simulink model "MySelectorCtrlMapping_RTW"  (R2022a)
settings: Solver=ode1  StartTime=0.0  StopTime=inf  FixedStep=0.001  RelTol=1e-3
PreLoadFcn:
  | vehicle = 'Car'; if ~length(which('cmself')), cmenv; end
  | MySelectorCtrlMapping_RTW_bus
InitFcn:
  | vehicle = 'Car'; if ~length(which('cmself')), cmenv; end
  | MySelectorCtrlMapping_RTW_bus
libraries: simulink x2
Description:
  | CarMaker Plug-in Model Target
settings Model: Creator=IPG  LastModifiedBy=IPG
settings DebuggingCC: UnconnectedInputMsg=warning  UnconnectedOutputMsg=warning  UnconnectedLineMsg=warning
settings RTWCC: Description=CarMaker Plug-in Model Target  SystemTargetFile=CarMaker.tlc  TemplateMakefile=CarMaker_unix-win64.tmf  DLArmComputeVersion=19.05
settings CodeAppCC: MaxIdLength=127
settings STFCustomTargetCC: TargetLangStandard=C99 (ISO)  CombineOutputUpdateFcns=on  MatFileLogging=on  CodeInterfacePackaging=Reusable function  GRTInterface=off  GenerateAllocFcn=on  SystemTargetFile=CarMaker.tlc
settings GRTTargetCC: ParMdlRefBuildCompliant=off  CompOptLevelCompliant=off  ConcurrentExecutionCompliant=off  CodeInterfacePackaging=Reusable function  CPPClassGenCompliant=off  GenerateAllocFcn=on  UseToolchainInfoCompliant=off

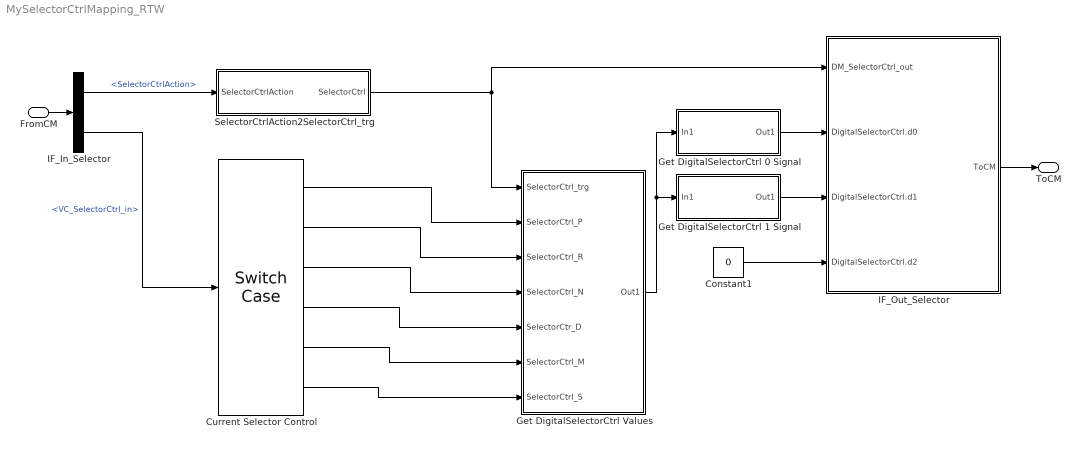
== system MySelectorCtrlMapping_RTW ==
  FromCM : Inport  OutDataTypeStr=Bus: cmSelectorCtrlMappingIn
  Constant1 : Constant  Value=0
  Current Selector Control : SwitchCase  CaseConditions={-9, -1, 0, 1, 2, 3}  ShowDefaultCase=off
  Get DigitalSelectorCtrl 0 Signal : Subsystem
  Get DigitalSelectorCtrl 1 Signal : Subsystem
  Get DigitalSelectorCtrl Values : Subsystem
  IF_In_Selector : BusSelector  OutputSignals=SelectorCtrlAction,VC_SelectorCtrl_in
  IF_Out_Selector : Subsystem  mask(Signal Selection){}
      mask help: Signal Selection Block
      settings: OpenFcn=cmSignalSelect('SignalSelection_CB',gcb)
  SelectorCtrlAction2SelectorCtrl_trg : Subsystem
  ToCM : Outport  OutDataTypeStr=Bus: cmSelectorCtrlMappingOut
  wires:
  FromCM/1 -> IF_In_Selector/1
  IF_Out_Selector/1(ToCM) -> ToCM/1
  Current Selector Control/6 -> Get DigitalSelectorCtrl Values/7(SelectorCtrl_S)
  IF_In_Selector/1 -> SelectorCtrlAction2SelectorCtrl_trg/1(SelectorCtrlAction)  "<SelectorCtrlAction>"
  Current Selector Control/2 -> Get DigitalSelectorCtrl Values/3(SelectorCtrl_R)
  Get DigitalSelectorCtrl 0 Signal/1(Out1) -> IF_Out_Selector/2(DigitalSelectorCtrl.d0)
  Get DigitalSelectorCtrl 1 Signal/1(Out1) -> IF_Out_Selector/3(DigitalSelectorCtrl.d1)
  Current Selector Control/3 -> Get DigitalSelectorCtrl Values/4(SelectorCtrl_N)
  SelectorCtrlAction2SelectorCtrl_trg/1(SelectorCtrl) -> IF_Out_Selector/1(DM_SelectorCtrl_out), Get DigitalSelectorCtrl Values/1(SelectorCtrl_trg)
  Current Selector Control/5 -> Get DigitalSelectorCtrl Values/6(SelectorCtrl_M)
  Current Selector Control/1 -> Get DigitalSelectorCtrl Values/2(SelectorCtrl_P)
  Constant1/1 -> IF_Out_Selector/4(DigitalSelectorCtrl.d2)
  Current Selector Control/4 -> Get DigitalSelectorCtrl Values/5(SelectorCtr_D)
  IF_In_Selector/2 -> Current Selector Control/1  "<VC_SelectorCtrl_in>"
  Get DigitalSelectorCtrl Values/1(Out1) -> Get DigitalSelectorCtrl 1 Signal/1(In1), Get DigitalSelectorCtrl 0 Signal/1(In1)

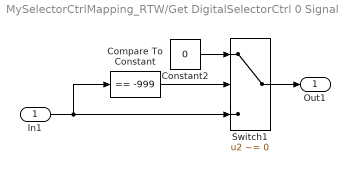
== system MySelectorCtrlMapping_RTW/Get DigitalSelectorCtrl 0 Signal ==
  In1 : Inport
  Compare To Constant : simulink/Logic and Bit Operations/Compare To Constant  relop===  const=-999  OutDataTypeStr=boolean
  Constant2 : Constant  Value=0
  Switch1 : Switch  Criteria=u2 ~= 0  SaturateOnIntegerOverflow=off  InputSameDT=off
  Out1 : Outport
  wires:
  Compare To Constant/1 -> Switch1/2
  Constant2/1 -> Switch1/1
  In1/1 -> Switch1/3, Compare To Constant/1
  Switch1/1 -> Out1/1

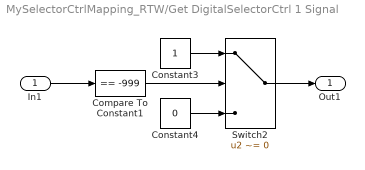
== system MySelectorCtrlMapping_RTW/Get DigitalSelectorCtrl 1 Signal ==
  In1 : Inport
  Compare To Constant1 : simulink/Logic and Bit Operations/Compare To Constant  relop===  const=-999  OutDataTypeStr=boolean
  Constant3 : Constant
  Constant4 : Constant  Value=0
  Switch2 : Switch  Criteria=u2 ~= 0  SaturateOnIntegerOverflow=off  InputSameDT=off
  Out1 : Outport
  wires:
  Compare To Constant1/1 -> Switch2/2
  Constant3/1 -> Switch2/1
  Constant4/1 -> Switch2/3
  In1/1 -> Compare To Constant1/1
  Switch2/1 -> Out1/1

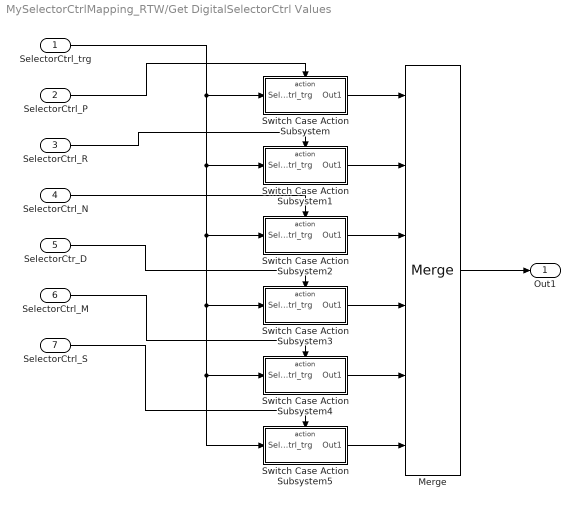
== system MySelectorCtrlMapping_RTW/Get DigitalSelectorCtrl Values ==
  SelectorCtrl_trg : Inport
  SelectorCtrl_P : Inport  Port=2
  SelectorCtrl_R : Inport  Port=3
  SelectorCtrl_N : Inport  Port=4
  SelectorCtr_D : Inport  Port=5
  SelectorCtrl_M : Inport  Port=6
  SelectorCtrl_S : Inport  Port=7
  Merge : Merge  Inputs=6
  Switch Case Action Subsystem : Subsystem  TreatAsAtomicUnit=on
  Switch Case Action Subsystem1 : Subsystem  TreatAsAtomicUnit=on
  Switch Case Action Subsystem2 : Subsystem  TreatAsAtomicUnit=on
  Switch Case Action Subsystem3 : Subsystem  TreatAsAtomicUnit=on
  Switch Case Action Subsystem4 : Subsystem  TreatAsAtomicUnit=on
  Switch Case Action Subsystem5 : Subsystem  TreatAsAtomicUnit=on
  Out1 : Outport
  wires:
  SelectorCtrl_trg/1 -> Switch Case Action Subsystem5/1(SelectorCtrl_trg), Switch Case Action Subsystem4/1(SelectorCtrl_trg), Switch Case Action Subsystem3/1(SelectorCtrl_trg), Switch Case Action Subsystem2/1(SelectorCtrl_trg), Switch Case Action Subsystem1/1(SelectorCtrl_trg), Switch Case Action Subsystem/1(SelectorCtrl_trg)
  SelectorCtrl_R/1 -> Switch Case Action Subsystem1/Action
  SelectorCtrl_N/1 -> Switch Case Action Subsystem2/Action
  SelectorCtrl_P/1 -> Switch Case Action Subsystem/Action
  SelectorCtr_D/1 -> Switch Case Action Subsystem3/Action
  SelectorCtrl_M/1 -> Switch Case Action Subsystem4/Action
  SelectorCtrl_S/1 -> Switch Case Action Subsystem5/Action
  Switch Case Action Subsystem/1(Out1) -> Merge/1
  Switch Case Action Subsystem1/1(Out1) -> Merge/2
  Switch Case Action Subsystem2/1(Out1) -> Merge/3
  Switch Case Action Subsystem3/1(Out1) -> Merge/4
  Switch Case Action Subsystem4/1(Out1) -> Merge/5
  Switch Case Action Subsystem5/1(Out1) -> Merge/6
  Merge/1 -> Out1/1

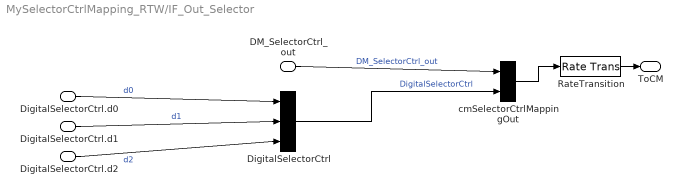
== system MySelectorCtrlMapping_RTW/IF_Out_Selector ==
  DM_SelectorCtrl_out : Inport
  DigitalSelectorCtrl.d0 : Inport  Port=2
  DigitalSelectorCtrl.d1 : Inport  Port=3
  DigitalSelectorCtrl.d2 : Inport  Port=4
  DigitalSelectorCtrl : BusCreator  Inputs=3
  RateTransition : RateTransition  OutPortSampleTime=str2num(get_param(bdroot,'FixedStep'))
  cmSelectorCtrlMappingOut : BusCreator  Inputs=2
  ToCM : Outport
  wires:
  RateTransition/1 -> ToCM/1
  cmSelectorCtrlMappingOut/1 -> RateTransition/1
  DigitalSelectorCtrl/1 -> cmSelectorCtrlMappingOut/2  "DigitalSelectorCtrl"
  DM_SelectorCtrl_out/1 -> cmSelectorCtrlMappingOut/1  "DM_SelectorCtrl_out"
  DigitalSelectorCtrl.d0/1 -> DigitalSelectorCtrl/1  "d0"
  DigitalSelectorCtrl.d1/1 -> DigitalSelectorCtrl/2  "d1"
  DigitalSelectorCtrl.d2/1 -> DigitalSelectorCtrl/3  "d2"

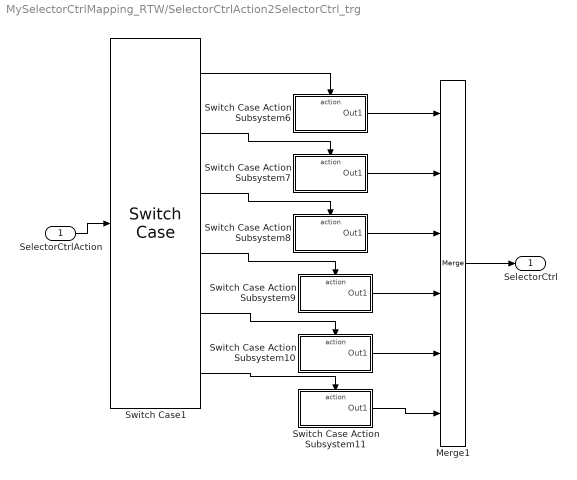
== system MySelectorCtrlMapping_RTW/SelectorCtrlAction2SelectorCtrl_trg ==
  SelectorCtrlAction : Inport
  Merge1 : Merge  Inputs=6
  Switch Case Action Subsystem10 : Subsystem  TreatAsAtomicUnit=on
  Switch Case Action Subsystem11 : Subsystem  TreatAsAtomicUnit=on
  Switch Case Action Subsystem6 : Subsystem  TreatAsAtomicUnit=on
  Switch Case Action Subsystem7 : Subsystem  TreatAsAtomicUnit=on
  Switch Case Action Subsystem8 : Subsystem  TreatAsAtomicUnit=on
  Switch Case Action Subsystem9 : Subsystem  TreatAsAtomicUnit=on
  Switch Case1 : SwitchCase  CaseConditions={0, 1, 2, 3, 4, 5}  ShowDefaultCase=off
  SelectorCtrl : Outport
  wires:
  Switch Case Action Subsystem9/1(Out1) -> Merge1/4
  Switch Case1/1 -> Switch Case Action Subsystem6/Action
  Switch Case1/3 -> Switch Case Action Subsystem8/Action
  Switch Case1/4 -> Switch Case Action Subsystem9/Action
  Switch Case1/2 -> Switch Case Action Subsystem7/Action
  Switch Case Action Subsystem7/1(Out1) -> Merge1/2
  Switch Case1/5 -> Switch Case Action Subsystem10/Action
  Switch Case Action Subsystem6/1(Out1) -> Merge1/1
  Switch Case Action Subsystem11/1(Out1) -> Merge1/6
  Switch Case Action Subsystem10/1(Out1) -> Merge1/5
  Switch Case Action Subsystem8/1(Out1) -> Merge1/3
  Switch Case1/6 -> Switch Case Action Subsystem11/Action
  SelectorCtrlAction/1 -> Switch Case1/1
  Merge1/1 -> SelectorCtrl/1

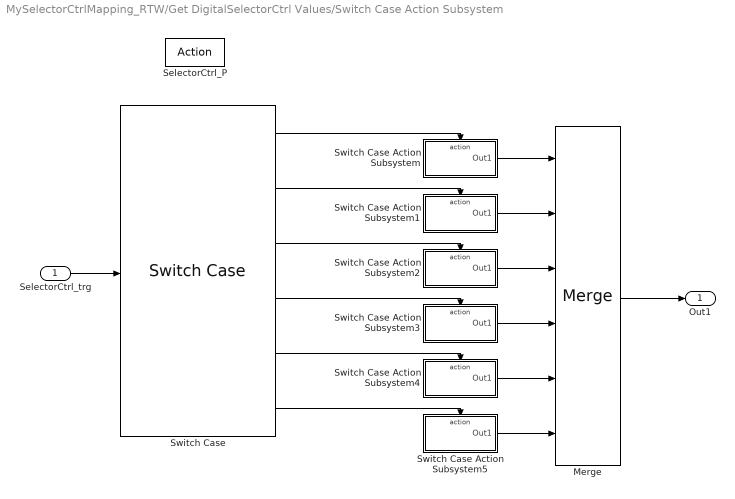
== system MySelectorCtrlMapping_RTW/Get DigitalSelectorCtrl Values/Switch Case Action Subsystem ==
  SelectorCtrl_trg : Inport
  SelectorCtrl_P : ActionPort
  Merge : Merge  Inputs=6
  Switch Case : SwitchCase  CaseConditions={-9,-1, 0, 1, 2, 3}  ShowDefaultCase=off
  Switch Case Action Subsystem : Subsystem  TreatAsAtomicUnit=on
  Switch Case Action Subsystem1 : Subsystem  TreatAsAtomicUnit=on
  Switch Case Action Subsystem2 : Subsystem  TreatAsAtomicUnit=on
  Switch Case Action Subsystem3 : Subsystem  TreatAsAtomicUnit=on
  Switch Case Action Subsystem4 : Subsystem  TreatAsAtomicUnit=on
  Switch Case Action Subsystem5 : Subsystem  TreatAsAtomicUnit=on
  Out1 : Outport
  wires:
  SelectorCtrl_trg/1 -> Switch Case/1
  Switch Case/1 -> Switch Case Action Subsystem/Action
  Merge/1 -> Out1/1
  Switch Case Action Subsystem/1(Out1) -> Merge/1
  Switch Case/2 -> Switch Case Action Subsystem1/Action
  Switch Case Action Subsystem1/1(Out1) -> Merge/2
  Switch Case/3 -> Switch Case Action Subsystem2/Action
  Switch Case/4 -> Switch Case Action Subsystem3/Action
  Switch Case/5 -> Switch Case Action Subsystem4/Action
  Switch Case/6 -> Switch Case Action Subsystem5/Action
  Switch Case Action Subsystem2/1(Out1) -> Merge/3
  Switch Case Action Subsystem3/1(Out1) -> Merge/4
  Switch Case Action Subsystem4/1(Out1) -> Merge/5
  Switch Case Action Subsystem5/1(Out1) -> Merge/6

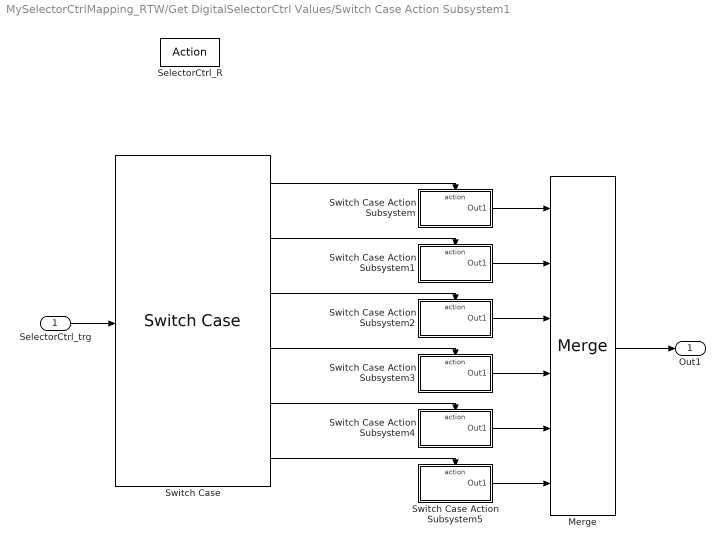
== system MySelectorCtrlMapping_RTW/Get DigitalSelectorCtrl Values/Switch Case Action Subsystem1 ==
  SelectorCtrl_trg : Inport
  SelectorCtrl_R : ActionPort
  Merge : Merge  Inputs=6
  Switch Case : SwitchCase  CaseConditions={-9,-1, 0, 1, 2, 3}  ShowDefaultCase=off
  Switch Case Action Subsystem : Subsystem  TreatAsAtomicUnit=on
  Switch Case Action Subsystem1 : Subsystem  TreatAsAtomicUnit=on
  Switch Case Action Subsystem2 : Subsystem  TreatAsAtomicUnit=on
  Switch Case Action Subsystem3 : Subsystem  TreatAsAtomicUnit=on
  Switch Case Action Subsystem4 : Subsystem  TreatAsAtomicUnit=on
  Switch Case Action Subsystem5 : Subsystem  TreatAsAtomicUnit=on
  Out1 : Outport
  wires:
  Switch Case Action Subsystem1/1(Out1) -> Merge/2
  Switch Case/5 -> Switch Case Action Subsystem4/Action
  Switch Case/3 -> Switch Case Action Subsystem2/Action
  SelectorCtrl_trg/1 -> Switch Case/1
  Switch Case/1 -> Switch Case Action Subsystem/Action
  Merge/1 -> Out1/1
  Switch Case Action Subsystem3/1(Out1) -> Merge/4
  Switch Case Action Subsystem4/1(Out1) -> Merge/5
  Switch Case/4 -> Switch Case Action Subsystem3/Action
  Switch Case/6 -> Switch Case Action Subsystem5/Action
  Switch Case Action Subsystem2/1(Out1) -> Merge/3
  Switch Case Action Subsystem5/1(Out1) -> Merge/6
  Switch Case Action Subsystem/1(Out1) -> Merge/1
  Switch Case/2 -> Switch Case Action Subsystem1/Action

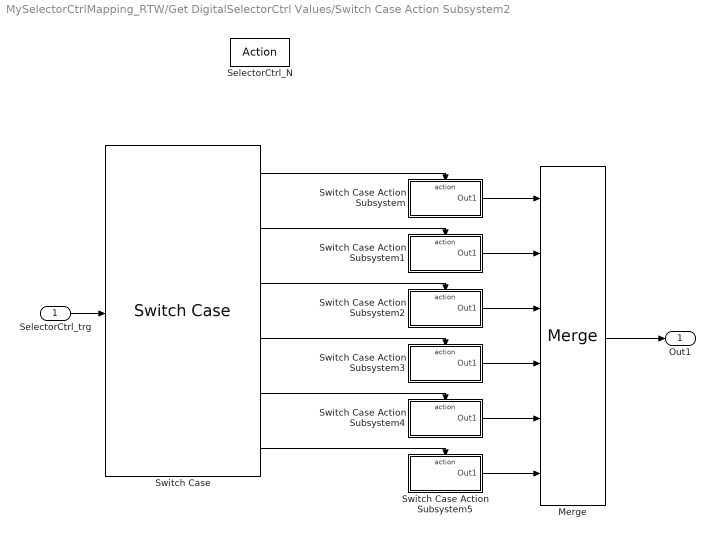
== system MySelectorCtrlMapping_RTW/Get DigitalSelectorCtrl Values/Switch Case Action Subsystem2 ==
  SelectorCtrl_trg : Inport
  SelectorCtrl_N : ActionPort
  Merge : Merge  Inputs=6
  Switch Case : SwitchCase  CaseConditions={-9,-1, 0, 1, 2, 3}  ShowDefaultCase=off
  Switch Case Action Subsystem : Subsystem  TreatAsAtomicUnit=on
  Switch Case Action Subsystem1 : Subsystem  TreatAsAtomicUnit=on
  Switch Case Action Subsystem2 : Subsystem  TreatAsAtomicUnit=on
  Switch Case Action Subsystem3 : Subsystem  TreatAsAtomicUnit=on
  Switch Case Action Subsystem4 : Subsystem  TreatAsAtomicUnit=on
  Switch Case Action Subsystem5 : Subsystem  TreatAsAtomicUnit=on
  Out1 : Outport
  wires:
  Switch Case/1 -> Switch Case Action Subsystem/Action
  Switch Case/6 -> Switch Case Action Subsystem5/Action
  Switch Case Action Subsystem2/1(Out1) -> Merge/3
  Switch Case/5 -> Switch Case Action Subsystem4/Action
  SelectorCtrl_trg/1 -> Switch Case/1
  Switch Case Action Subsystem1/1(Out1) -> Merge/2
  Switch Case Action Subsystem5/1(Out1) -> Merge/6
  Switch Case Action Subsystem4/1(Out1) -> Merge/5
  Switch Case/4 -> Switch Case Action Subsystem3/Action
  Switch Case/2 -> Switch Case Action Subsystem1/Action
  Switch Case Action Subsystem3/1(Out1) -> Merge/4
  Switch Case Action Subsystem/1(Out1) -> Merge/1
  Switch Case/3 -> Switch Case Action Subsystem2/Action
  Merge/1 -> Out1/1

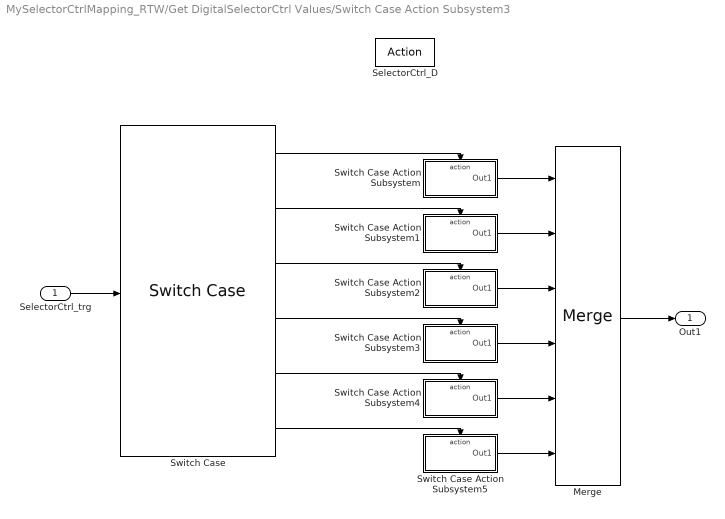
== system MySelectorCtrlMapping_RTW/Get DigitalSelectorCtrl Values/Switch Case Action Subsystem3 ==
  SelectorCtrl_trg : Inport
  SelectorCtrl_D : ActionPort
  Merge : Merge  Inputs=6
  Switch Case : SwitchCase  CaseConditions={-9,-1, 0, 1, 2, 3}  ShowDefaultCase=off
  Switch Case Action Subsystem : Subsystem  TreatAsAtomicUnit=on
  Switch Case Action Subsystem1 : Subsystem  TreatAsAtomicUnit=on
  Switch Case Action Subsystem2 : Subsystem  TreatAsAtomicUnit=on
  Switch Case Action Subsystem3 : Subsystem  TreatAsAtomicUnit=on
  Switch Case Action Subsystem4 : Subsystem  TreatAsAtomicUnit=on
  Switch Case Action Subsystem5 : Subsystem  TreatAsAtomicUnit=on
  Out1 : Outport
  wires:
  Switch Case Action Subsystem2/1(Out1) -> Merge/3
  Switch Case Action Subsystem1/1(Out1) -> Merge/2
  Switch Case/5 -> Switch Case Action Subsystem4/Action
  Switch Case Action Subsystem/1(Out1) -> Merge/1
  Switch Case/4 -> Switch Case Action Subsystem3/Action
  Switch Case/2 -> Switch Case Action Subsystem1/Action
  SelectorCtrl_trg/1 -> Switch Case/1
  Switch Case Action Subsystem3/1(Out1) -> Merge/4
  Switch Case/1 -> Switch Case Action Subsystem/Action
  Switch Case Action Subsystem5/1(Out1) -> Merge/6
  Switch Case Action Subsystem4/1(Out1) -> Merge/5
  Switch Case/6 -> Switch Case Action Subsystem5/Action
  Merge/1 -> Out1/1
  Switch Case/3 -> Switch Case Action Subsystem2/Action

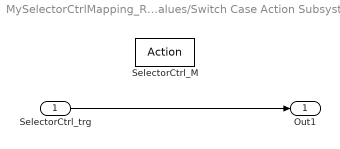
== system MySelectorCtrlMapping_RTW/Get DigitalSelectorCtrl Values/Switch Case Action Subsystem4 ==
  SelectorCtrl_trg : Inport
  SelectorCtrl_M : ActionPort
  Out1 : Outport
  wires:
  SelectorCtrl_trg/1 -> Out1/1

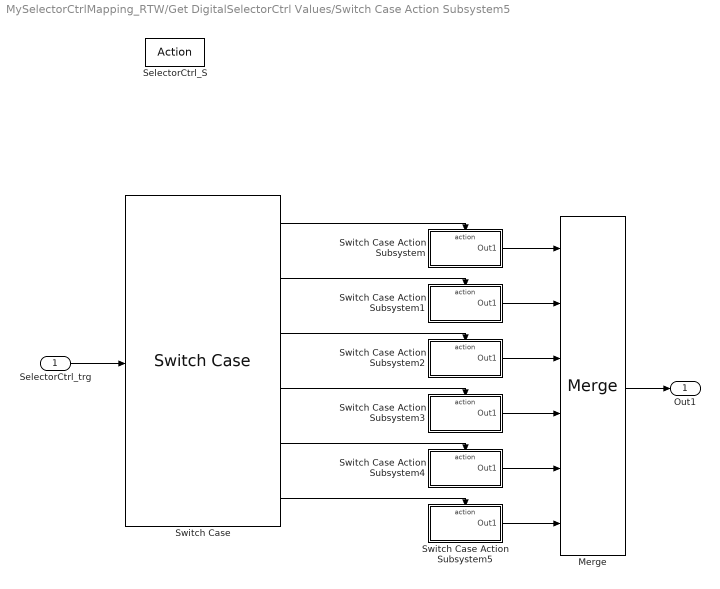
== system MySelectorCtrlMapping_RTW/Get DigitalSelectorCtrl Values/Switch Case Action Subsystem5 ==
  SelectorCtrl_trg : Inport
  SelectorCtrl_S : ActionPort
  Merge : Merge  Inputs=6
  Switch Case : SwitchCase  CaseConditions={-9,-1, 0, 1, 2, 3}  ShowDefaultCase=off
  Switch Case Action Subsystem : Subsystem  TreatAsAtomicUnit=on
  Switch Case Action Subsystem1 : Subsystem  TreatAsAtomicUnit=on
  Switch Case Action Subsystem2 : Subsystem  TreatAsAtomicUnit=on
  Switch Case Action Subsystem3 : Subsystem  TreatAsAtomicUnit=on
  Switch Case Action Subsystem4 : Subsystem  TreatAsAtomicUnit=on
  Switch Case Action Subsystem5 : Subsystem  TreatAsAtomicUnit=on
  Out1 : Outport
  wires:
  Switch Case Action Subsystem2/1(Out1) -> Merge/3
  Switch Case/5 -> Switch Case Action Subsystem4/Action
  Switch Case Action Subsystem3/1(Out1) -> Merge/4
  Switch Case Action Subsystem5/1(Out1) -> Merge/6
  Merge/1 -> Out1/1
  Switch Case Action Subsystem/1(Out1) -> Merge/1
  Switch Case/2 -> Switch Case Action Subsystem1/Action
  Switch Case/3 -> Switch Case Action Subsystem2/Action
  Switch Case/1 -> Switch Case Action Subsystem/Action
  Switch Case/6 -> Switch Case Action Subsystem5/Action
  Switch Case Action Subsystem4/1(Out1) -> Merge/5
  Switch Case/4 -> Switch Case Action Subsystem3/Action
  Switch Case Action Subsystem1/1(Out1) -> Merge/2
  SelectorCtrl_trg/1 -> Switch Case/1

== system MySelectorCtrlMapping_RTW/SelectorCtrlAction2SelectorCtrl_trg/Switch Case Action Subsystem10 ==
  Action Port : ActionPort
  Constant : Constant  Value=-1
  Out1 : Outport
  wires:
  Constant/1 -> Out1/1

== system MySelectorCtrlMapping_RTW/SelectorCtrlAction2SelectorCtrl_trg/Switch Case Action Subsystem11 ==
  Action Port : ActionPort
  Constant : Constant  Value=3
  Out1 : Outport
  wires:
  Constant/1 -> Out1/1

== system MySelectorCtrlMapping_RTW/SelectorCtrlAction2SelectorCtrl_trg/Switch Case Action Subsystem6 ==
  Action Port : ActionPort
  Constant : Constant  Value=-9999
  Out1 : Outport
  wires:
  Constant/1 -> Out1/1

== system MySelectorCtrlMapping_RTW/SelectorCtrlAction2SelectorCtrl_trg/Switch Case Action Subsystem7 ==
  Action Port : ActionPort
  Constant : Constant  Value=0
  Out1 : Outport
  wires:
  Constant/1 -> Out1/1

== system MySelectorCtrlMapping_RTW/SelectorCtrlAction2SelectorCtrl_trg/Switch Case Action Subsystem8 ==
  Action Port : ActionPort
  Constant : Constant  Value=-9
  Out1 : Outport
  wires:
  Constant/1 -> Out1/1

== system MySelectorCtrlMapping_RTW/SelectorCtrlAction2SelectorCtrl_trg/Switch Case Action Subsystem9 ==
  Action Port : ActionPort
  Constant : Constant
  Out1 : Outport
  wires:
  Constant/1 -> Out1/1

== system MySelectorCtrlMapping_RTW/Get DigitalSelectorCtrl Values/Switch Case Action Subsystem/Switch Case Action Subsystem ==
  Action Port : ActionPort
  Constant : Constant  Value=0
  Out1 : Outport
  wires:
  Constant/1 -> Out1/1

== system MySelectorCtrlMapping_RTW/Get DigitalSelectorCtrl Values/Switch Case Action Subsystem/Switch Case Action Subsystem1 ==
  Action Port : ActionPort
  Constant : Constant  Value=2
  Out1 : Outport
  wires:
  Constant/1 -> Out1/1

== system MySelectorCtrlMapping_RTW/Get DigitalSelectorCtrl Values/Switch Case Action Subsystem/Switch Case Action Subsystem2 ==
  Action Port : ActionPort
  Constant : Constant
  Out1 : Outport
  wires:
  Constant/1 -> Out1/1

== system MySelectorCtrlMapping_RTW/Get DigitalSelectorCtrl Values/Switch Case Action Subsystem/Switch Case Action Subsystem3 ==
  Action Port : ActionPort
  Constant : Constant
  Out1 : Outport
  wires:
  Constant/1 -> Out1/1

== system MySelectorCtrlMapping_RTW/Get DigitalSelectorCtrl Values/Switch Case Action Subsystem/Switch Case Action Subsystem4 ==
  Action Port : ActionPort
  Constant : Constant  Value=3
  Out1 : Outport
  wires:
  Constant/1 -> Out1/1

== system MySelectorCtrlMapping_RTW/Get DigitalSelectorCtrl Values/Switch Case Action Subsystem/Switch Case Action Subsystem5 ==
  Action Port : ActionPort
  Constant : Constant  Value=2
  Out1 : Outport
  wires:
  Constant/1 -> Out1/1

== system MySelectorCtrlMapping_RTW/Get DigitalSelectorCtrl Values/Switch Case Action Subsystem1/Switch Case Action Subsystem ==
  Action Port : ActionPort
  Constant : Constant  Value=-999
  Out1 : Outport
  wires:
  Constant/1 -> Out1/1

== system MySelectorCtrlMapping_RTW/Get DigitalSelectorCtrl Values/Switch Case Action Subsystem1/Switch Case Action Subsystem1 ==
  Action Port : ActionPort
  Constant : Constant  Value=0
  Out1 : Outport
  wires:
  Constant/1 -> Out1/1

== system MySelectorCtrlMapping_RTW/Get DigitalSelectorCtrl Values/Switch Case Action Subsystem1/Switch Case Action Subsystem2 ==
  Action Port : ActionPort
  Constant : Constant  Value=-1
  Out1 : Outport
  wires:
  Constant/1 -> Out1/1

== system MySelectorCtrlMapping_RTW/Get DigitalSelectorCtrl Values/Switch Case Action Subsystem1/Switch Case Action Subsystem3 ==
  Action Port : ActionPort
  Constant : Constant  Value=-2
  Out1 : Outport
  wires:
  Constant/1 -> Out1/1

== system MySelectorCtrlMapping_RTW/Get DigitalSelectorCtrl Values/Switch Case Action Subsystem1/Switch Case Action Subsystem4 ==
  Action Port : ActionPort
  Constant : Constant  Value=3
  Out1 : Outport
  wires:
  Constant/1 -> Out1/1

== system MySelectorCtrlMapping_RTW/Get DigitalSelectorCtrl Values/Switch Case Action Subsystem1/Switch Case Action Subsystem5 ==
  Action Port : ActionPort
  Constant : Constant  Value=3
  Out1 : Outport
  wires:
  Constant/1 -> Out1/1

== system MySelectorCtrlMapping_RTW/Get DigitalSelectorCtrl Values/Switch Case Action Subsystem2/Switch Case Action Subsystem ==
  Action Port : ActionPort
  Constant : Constant  Value=-999
  Out1 : Outport
  wires:
  Constant/1 -> Out1/1

== system MySelectorCtrlMapping_RTW/Get DigitalSelectorCtrl Values/Switch Case Action Subsystem2/Switch Case Action Subsystem1 ==
  Action Port : ActionPort
  Constant : Constant
  Out1 : Outport
  wires:
  Constant/1 -> Out1/1

== system MySelectorCtrlMapping_RTW/Get DigitalSelectorCtrl Values/Switch Case Action Subsystem2/Switch Case Action Subsystem2 ==
  Action Port : ActionPort
  Constant : Constant  Value=0
  Out1 : Outport
  wires:
  Constant/1 -> Out1/1

== system MySelectorCtrlMapping_RTW/Get DigitalSelectorCtrl Values/Switch Case Action Subsystem2/Switch Case Action Subsystem3 ==
  Action Port : ActionPort
  Constant : Constant  Value=-1
  Out1 : Outport
  wires:
  Constant/1 -> Out1/1

== system MySelectorCtrlMapping_RTW/Get DigitalSelectorCtrl Values/Switch Case Action Subsystem2/Switch Case Action Subsystem4 ==
  Action Port : ActionPort
  Constant : Constant  Value=3
  Out1 : Outport
  wires:
  Constant/1 -> Out1/1

== system MySelectorCtrlMapping_RTW/Get DigitalSelectorCtrl Values/Switch Case Action Subsystem2/Switch Case Action Subsystem5 ==
  Action Port : ActionPort
  Constant : Constant  Value=-2
  Out1 : Outport
  wires:
  Constant/1 -> Out1/1

== system MySelectorCtrlMapping_RTW/Get DigitalSelectorCtrl Values/Switch Case Action Subsystem3/Switch Case Action Subsystem ==
  Action Port : ActionPort
  Constant : Constant  Value=-999
  Out1 : Outport
  wires:
  Constant/1 -> Out1/1

== system MySelectorCtrlMapping_RTW/Get DigitalSelectorCtrl Values/Switch Case Action Subsystem3/Switch Case Action Subsystem1 ==
  Action Port : ActionPort
  Constant : Constant  Value=2
  Out1 : Outport
  wires:
  Constant/1 -> Out1/1

== system MySelectorCtrlMapping_RTW/Get DigitalSelectorCtrl Values/Switch Case Action Subsystem3/Switch Case Action Subsystem2 ==
  Action Port : ActionPort
  Constant : Constant
  Out1 : Outport
  wires:
  Constant/1 -> Out1/1

== system MySelectorCtrlMapping_RTW/Get DigitalSelectorCtrl Values/Switch Case Action Subsystem3/Switch Case Action Subsystem3 ==
  Action Port : ActionPort
  Constant : Constant  Value=0
  Out1 : Outport
  wires:
  Constant/1 -> Out1/1

== system MySelectorCtrlMapping_RTW/Get DigitalSelectorCtrl Values/Switch Case Action Subsystem3/Switch Case Action Subsystem4 ==
  Action Port : ActionPort
  Constant : Constant  Value=3
  Out1 : Outport
  wires:
  Constant/1 -> Out1/1

== system MySelectorCtrlMapping_RTW/Get DigitalSelectorCtrl Values/Switch Case Action Subsystem3/Switch Case Action Subsystem5 ==
  Action Port : ActionPort
  Constant : Constant  Value=-1
  Out1 : Outport
  wires:
  Constant/1 -> Out1/1

== system MySelectorCtrlMapping_RTW/Get DigitalSelectorCtrl Values/Switch Case Action Subsystem5/Switch Case Action Subsystem ==
  Action Port : ActionPort
  Constant : Constant  Value=-999
  Out1 : Outport
  wires:
  Constant/1 -> Out1/1

== system MySelectorCtrlMapping_RTW/Get DigitalSelectorCtrl Values/Switch Case Action Subsystem5/Switch Case Action Subsystem1 ==
  Action Port : ActionPort
  Constant : Constant  Value=2
  Out1 : Outport
  wires:
  Constant/1 -> Out1/1

== system MySelectorCtrlMapping_RTW/Get DigitalSelectorCtrl Values/Switch Case Action Subsystem5/Switch Case Action Subsystem2 ==
  Action Port : ActionPort
  Constant : Constant
  Out1 : Outport
  wires:
  Constant/1 -> Out1/1

== system MySelectorCtrlMapping_RTW/Get DigitalSelectorCtrl Values/Switch Case Action Subsystem5/Switch Case Action Subsystem3 ==
  Action Port : ActionPort
  Constant : Constant  Value=-1
  Out1 : Outport
  wires:
  Constant/1 -> Out1/1

== system MySelectorCtrlMapping_RTW/Get DigitalSelectorCtrl Values/Switch Case Action Subsystem5/Switch Case Action Subsystem4 ==
  Action Port : ActionPort
  Constant : Constant  Value=3
  Out1 : Outport
  wires:
  Constant/1 -> Out1/1

== system MySelectorCtrlMapping_RTW/Get DigitalSelectorCtrl Values/Switch Case Action Subsystem5/Switch Case Action Subsystem5 ==
  Action Port : ActionPort
  Constant : Constant  Value=0
  Out1 : Outport
  wires:
  Constant/1 -> Out1/1
